simulink model "prelab6bModel"  (R2016b)
settings: Solver=VariableStepAuto  StartTime=0.0  StopTime=10.0  RelTol=1e-3
values from neighbouring files (symbols this model uses):
  A = [ 0 a12  0   0 ... (first row only)    [ee128lab6b.m]
  B = [0 b2 0 b4]'    [ee128lab6b.m]
  C = [1 0 0 0]    [ee128lab6b.m]
  K = acker(A,B, [-2+10*j,-2-10*j,-1.6+1.3*j, -1.6-1.3*j])    [ee128lab6b.m]
  L = (place(A' ,C', [-10+15*1i -10-15*1i -12+17*1i -12-17*1i]))'    [ee128lab6b.m]
settings Model: Creator=juanrodriguezquintanilla  LastModifiedBy=juanrodriguezquintanilla
settings DataIOCC: SaveFormat=Array  SaveOutput=off  SaveState=on  OutputSaveName=mierda

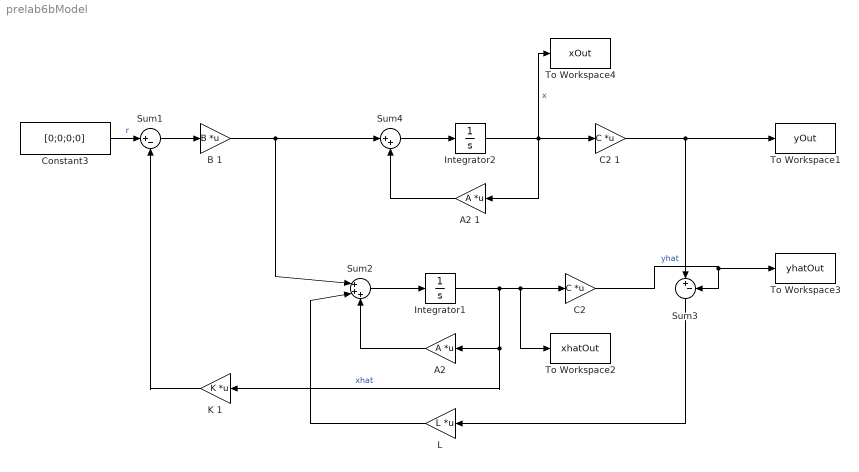
== system prelab6bModel ==
  "A2 " : Gain  Gain=A  Multiplication=Matrix(K*u)
  A2 1 : Gain  Gain=A  Multiplication=Matrix(K*u)
  B 1 : Gain  Gain=B  Multiplication=Matrix(K*u)
  "C2 " : Gain  Gain=C  Multiplication=Matrix(K*u)
  C2 1 : Gain  Gain=C  Multiplication=Matrix(K*u)
  Constant3 : Constant  Value=[0;0;0;0]
  Integrator1 : Integrator
  Integrator2 : Integrator
  K 1 : Gain  Gain=K  Multiplication=Matrix(K*u)
  "L " : Gain  Gain=L  Multiplication=Matrix(K*u)
  Sum1 : Sum  Inputs=|+-
  Sum2 : Sum  Inputs=|+++
  Sum3 : Sum  Inputs=|+-
  Sum4 : Sum  Inputs=|++
  To Workspace1 : ToWorkspace  VariableName=yOut  SaveFormat=Timeseries  SampleTime=-1
      settings: MaxDataPoints=100
  To Workspace2 : ToWorkspace  VariableName=xhatOut  SaveFormat=Timeseries  SampleTime=-1
  To Workspace3 : ToWorkspace  VariableName=yhatOut  SaveFormat=Timeseries  SampleTime=-1
      settings: MaxDataPoints=100
  To Workspace4 : ToWorkspace  VariableName=xOut  SaveFormat=Timeseries  SampleTime=-1
  wires:
  Constant3/1 -> Sum1/1  "r"
  Sum2/1 -> Integrator1/1
  Integrator1/1 -> K 1/1, "A2 "/1, "C2 "/1, To Workspace2/1  "xhat"
  "C2 "/1 -> To Workspace3/1, Sum3/2  "yhat"
  Sum3/1 -> "L "/1
  "A2 "/1 -> Sum2/3
  "L "/1 -> Sum2/2
  Sum1/1 -> B 1/1
  K 1/1 -> Sum1/2
  Sum4/1 -> Integrator2/1
  Integrator2/1 -> To Workspace4/1, C2 1/1, A2 1/1  "x"
  A2 1/1 -> Sum4/2
  C2 1/1 -> To Workspace1/1, Sum3/1
  B 1/1 -> Sum2/1, Sum4/1
